simulink model "wheelspeed"  (R2020a)
settings: Solver=ode45  StartTime=0.0  StopTime=25  MaxStep=0.01  RelTol=1e-3  AbsTol=1e-6
values from neighbouring files (symbols this model uses):
  ctrl = 1    [abs.mat]
  g = 32.18    [abs.mat]
  m = 50    [abs.mat]
  mu = [0 0.4 0.8 0.97 1 0.98 0.96 0.94 0.92 0.9 0.88 0.855 ... (21 elements, 1x21)]    [abs.mat]
  Rr = 1.25    [abs.mat]
  slip = [0 0.05 0.1 0.15 0.2 0.25 0.3 0.35 0.4 0.45 0.5 0.55 ... (21 elements, 1x21)]    [abs.mat]
  v0 = 88    [abs.mat]
settings Model: Creator=Admin  LastModifiedBy=Admin
settings SolverCC: AutoScaleAbsTol=off

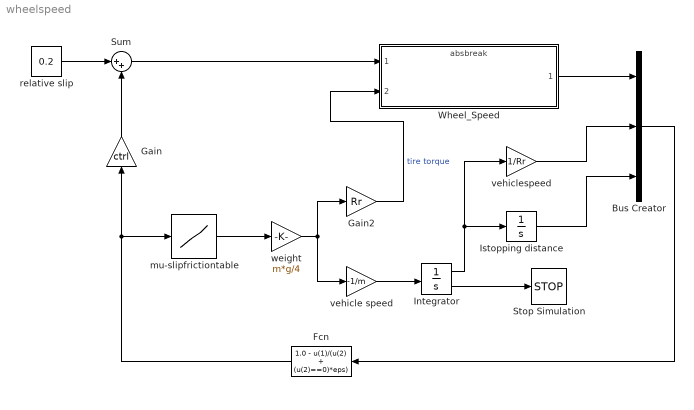
== system wheelspeed ==
  Bus Creator : BusCreator  Inputs=3
  Fcn : Fcn  Expr=1.0 - u(1)/(u(2) + (u(2)==0)*eps)
  Gain : Gain  Gain=ctrl
  Gain2 : Gain  Gain=Rr
  Integrator : Integrator  InitialCondition=v0  LimitOutput=on  UpperSaturationLimit=1000  LowerSaturationLimit=0  ShowSaturationPort=on
  Istopping distance : Integrator
  Stop Simulation : Stop
  Sum : Sum  Inputs=|++
  Wheel_Speed : ModelReference  ModelNameDialog=absbreak.slx  ModelReferenceVersion=1.3
  mu-slipfrictiontable : Lookup_n-D  NumberOfTableDimensions=1  BreakpointsForDimension1=slip  Table=mu  InternalRulePriority=Speed  RndMeth=Simplest  InputSameDT=on
  relative slip : Constant  Value=0.2
  vehicle speed : Gain  Gain=-1/m
  vehiclespeed : Gain  Gain=1/Rr
  weight : Gain  Gain=m*g/4
  wires:
  Gain2/1 -> Wheel_Speed/2  "tire torque"
  Wheel_Speed/1 -> Bus Creator/1
  Sum/1 -> Wheel_Speed/1
  relative slip/1 -> Sum/1
  Gain/1 -> Sum/2
  mu-slipfrictiontable/1 -> weight/1
  weight/1 -> vehicle speed/1, Gain2/1
  vehicle speed/1 -> Integrator/1
  Integrator/1 -> vehiclespeed/1, Istopping distance/1
  vehiclespeed/1 -> Bus Creator/2
  Istopping distance/1 -> Bus Creator/3
  Bus Creator/1 -> Fcn/1
  Fcn/1 -> Gain/1, mu-slipfrictiontable/1
  Integrator/2 -> Stop Simulation/1
